simulink library "Teleop_lib"  (R2023b)
settings: Solver=VariableStepAuto  StartTime=0.0  StopTime=10.0  RelTol=1e-3
undefined symbols (not defined in the file): Spline_Num_Poses_default, Spline_Ref_Poses_default, TEST_Swerve_Mode_Override_Flag
settings Model: Creator=FIRSTMentor  LastModifiedBy=ander

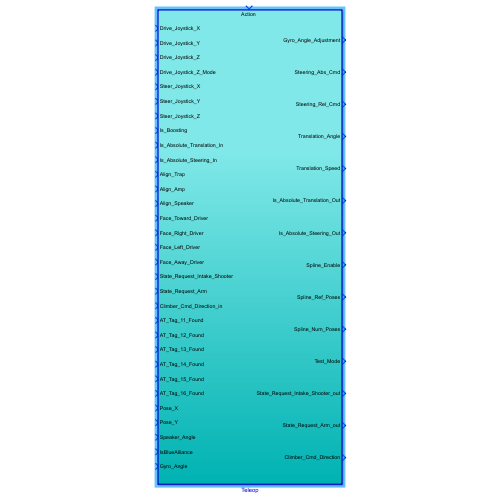
[thumbnail: Simulink's stored preview of the top-level diagram]
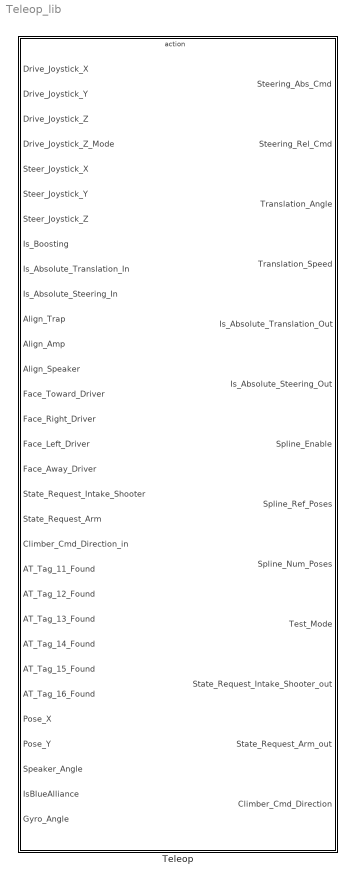
== system Teleop_lib ==
  Teleop : Subsystem  TreatAsAtomicUnit=on

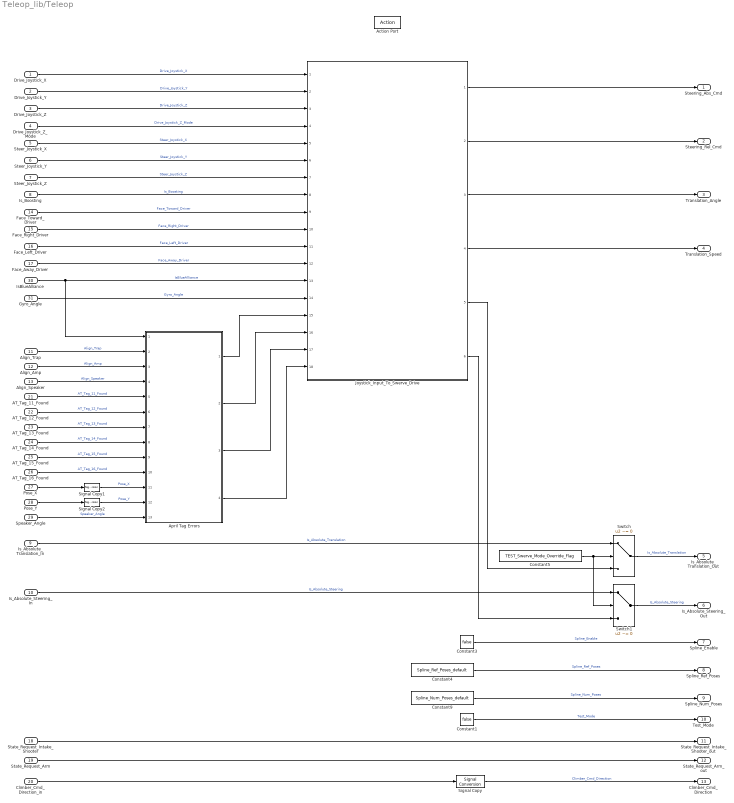
== system Teleop_lib/Teleop ==
  Drive_Joystick_X : Inport
  Drive_Joystick_Y : Inport  Port=2
  Drive_Joystick_Z : Inport  Port=3
  Drive_Joystick_Z_Mode : Inport  Port=4
  Steer_Joystick_X : Inport  Port=5
  Steer_Joystick_Y : Inport  Port=6
  Steer_Joystick_Z : Inport  Port=7
  Is_Boosting : Inport  Port=8
  Is_Absolute_Translation_In : Inport  Port=9
  Is_Absolute_Steering_In : Inport  Port=10
  Align_Trap : Inport  Port=11
  Align_Amp : Inport  Port=12
  Align_Speaker : Inport  Port=13
  Face_Toward_Driver : Inport  Port=14
  Face_Right_Driver : Inport  Port=15
  Face_Left_Driver : Inport  Port=16
  Face_Away_Driver : Inport  Port=17
  State_Request_Intake_Shooter : Inport  Port=18
  State_Request_Arm : Inport  Port=19
  Climber_Cmd_Direction_in : Inport  Port=20
  AT_Tag_11_Found : Inport  Port=21
  AT_Tag_12_Found : Inport  Port=22
  AT_Tag_13_Found : Inport  Port=23
  AT_Tag_14_Found : Inport  Port=24
  AT_Tag_15_Found : Inport  Port=25
  AT_Tag_16_Found : Inport  Port=26
  Pose_X : Inport  Port=27
  Pose_Y : Inport  Port=28
  Speaker_Angle : Inport  Port=29
  IsBlueAlliance : Inport  Port=30
  Gyro_Angle : Inport  Port=31
  Action Port : ActionPort
  April Tag Errors : Subsystem  ReferencedSubsystem=April_Tag_Errors
  Constant1 : Constant  Value=false  OutDataTypeStr=boolean
  Constant3 : Constant  Value=false  OutDataTypeStr=boolean
  Constant4 : Constant  Value=Spline_Ref_Poses_default
  Constant5 : Constant  Value=TEST_Swerve_Mode_Override_Flag
  Constant9 : Constant  Value=Spline_Num_Poses_default  OutDataTypeStr=double
  Joystick_Input_To_Swerve_Drive : Subsystem  ReferencedSubsystem=Joystick_Input_To_Swerve_Drive_sub
  Signal Copy : SignalConversion  OverrideOpt=off
  Signal Copy1 : SignalConversion  OverrideOpt=off
  Signal Copy2 : SignalConversion  OverrideOpt=off
  Switch : Switch  Criteria=u2 ~= 0  SaturateOnIntegerOverflow=off  InputSameDT=off
  Switch1 : Switch  Criteria=u2 ~= 0  SaturateOnIntegerOverflow=off  InputSameDT=off
  Steering_Abs_Cmd : Outport
  Steering_Rel_Cmd : Outport  Port=2
  Translation_Angle : Outport  Port=3
  Translation_Speed : Outport  Port=4
  Is_Absolute_Translation_Out : Outport  Port=5
  Is_Absolute_Steering_Out : Outport  Port=6
  Spline_Enable : Outport  Port=7
  Spline_Ref_Poses : Outport  Port=8
  Spline_Num_Poses : Outport  Port=9
  Test_Mode : Outport  Port=10
  State_Request_Intake_Shooter_out : Outport  Port=11
  State_Request_Arm_out : Outport  Port=12
  Climber_Cmd_Direction : Outport  Port=13
  wires:
  Steer_Joystick_X/1 -> Joystick_Input_To_Swerve_Drive/5  "Steer_Joystick_X"
  Steer_Joystick_Y/1 -> Joystick_Input_To_Swerve_Drive/6  "Steer_Joystick_Y"
  Drive_Joystick_X/1 -> Joystick_Input_To_Swerve_Drive/1  "Drive_Joystick_X"
  Drive_Joystick_Y/1 -> Joystick_Input_To_Swerve_Drive/2  "Drive_Joystick_Y"
  Joystick_Input_To_Swerve_Drive/1 -> Steering_Abs_Cmd/1
  Joystick_Input_To_Swerve_Drive/2 -> Steering_Rel_Cmd/1
  Joystick_Input_To_Swerve_Drive/3 -> Translation_Angle/1
  Joystick_Input_To_Swerve_Drive/4 -> Translation_Speed/1
  Switch1/1 -> Is_Absolute_Steering_Out/1  "Is_Absolute_Steering"
  Is_Boosting/1 -> Joystick_Input_To_Swerve_Drive/8  "Is_Boosting"
  Constant9/1 -> Spline_Num_Poses/1  "Spline_Num_Poses"
  Constant4/1 -> Spline_Ref_Poses/1  "Spline_Ref_Poses"
  Constant3/1 -> Spline_Enable/1  "Spline_Enable"
  Constant1/1 -> Test_Mode/1  "Test_Mode"
  State_Request_Intake_Shooter/1 -> State_Request_Intake_Shooter_out/1
  State_Request_Arm/1 -> State_Request_Arm_out/1
  Drive_Joystick_Z/1 -> Joystick_Input_To_Swerve_Drive/3  "Drive_Joystick_Z"
  Steer_Joystick_Z/1 -> Joystick_Input_To_Swerve_Drive/7  "Steer_Joystick_Z"
  Face_Toward_Driver/1 -> Joystick_Input_To_Swerve_Drive/9  "Face_Toward_Driver"
  Face_Right_Driver/1 -> Joystick_Input_To_Swerve_Drive/10  "Face_Right_Driver"
  Face_Left_Driver/1 -> Joystick_Input_To_Swerve_Drive/11  "Face_Left_Driver"
  Face_Away_Driver/1 -> Joystick_Input_To_Swerve_Drive/12  "Face_Away_Driver"
  Climber_Cmd_Direction_in/1 -> Signal Copy/1
  Signal Copy/1 -> Climber_Cmd_Direction/1  "Climber_Cmd_Direction"
  Is_Absolute_Steering_In/1 -> Switch1/1  "Is_Absolute_Steering"
  Constant5/1 -> Switch/2, Switch1/2
  Switch/1 -> Is_Absolute_Translation_Out/1  "Is_Absolute_Translation"
  Is_Absolute_Translation_In/1 -> Switch/1  "Is_Absolute_Translation"
  Joystick_Input_To_Swerve_Drive/5 -> Switch/3
  Pose_X/1 -> Signal Copy1/1
  Pose_Y/1 -> Signal Copy2/1
  April Tag Errors/2 -> Joystick_Input_To_Swerve_Drive/16
  April Tag Errors/3 -> Joystick_Input_To_Swerve_Drive/17
  April Tag Errors/4 -> Joystick_Input_To_Swerve_Drive/18
  IsBlueAlliance/1 -> Joystick_Input_To_Swerve_Drive/13, April Tag Errors/1  "IsBlueAlliance"
  Drive_Joystick_Z_Mode/1 -> Joystick_Input_To_Swerve_Drive/4  "Drive_Joystick_Z_Mode"
  Joystick_Input_To_Swerve_Drive/6 -> Switch1/3
  Gyro_Angle/1 -> Joystick_Input_To_Swerve_Drive/14  "Gyro_Angle"
  Align_Trap/1 -> April Tag Errors/2  "Align_Trap"
  Align_Amp/1 -> April Tag Errors/3  "Align_Amp"
  Align_Speaker/1 -> April Tag Errors/4  "Align_Speaker"
  AT_Tag_11_Found/1 -> April Tag Errors/5  "AT_Tag_11_Found"
  AT_Tag_12_Found/1 -> April Tag Errors/6  "AT_Tag_12_Found"
  AT_Tag_13_Found/1 -> April Tag Errors/7  "AT_Tag_13_Found"
  AT_Tag_14_Found/1 -> April Tag Errors/8  "AT_Tag_14_Found"
  AT_Tag_15_Found/1 -> April Tag Errors/9  "AT_Tag_15_Found"
  AT_Tag_16_Found/1 -> April Tag Errors/10  "AT_Tag_16_Found"
  Signal Copy1/1 -> April Tag Errors/11  "Pose_X"
  Signal Copy2/1 -> April Tag Errors/12  "Pose_Y"
  Speaker_Angle/1 -> April Tag Errors/13  "Speaker_Angle"
  April Tag Errors/1 -> Joystick_Input_To_Swerve_Drive/15
